simulink model "noisefilterfunction"  (Simulink 7.7)
settings: Solver=ode45  StartTime=0.0  StopTime=1000  RelTol=1e-3
settings Model: Creator=kevin  LastModifiedBy=kevin

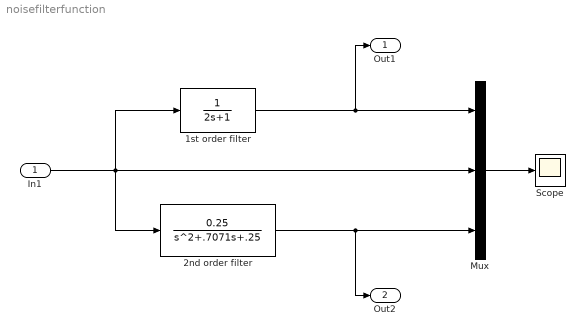
== system noisefilterfunction ==
  In1 : Inport
  1st order filter : TransferFcn  Denominator=[2 1]
  2nd order filter : TransferFcn  Numerator=[0.25]  Denominator=[1 .7071 .25]
  Mux : Mux  Inputs=3
  Scope : Scope
      settings: TimeRange=500  YMin=-4  YMax=4
  Out1 : Outport
  Out2 : Outport  Port=2
  wires:
  2nd order filter/1 -> Mux/3, Out2/1
  1st order filter/1 -> Mux/1, Out1/1
  In1/1 -> Mux/2, 1st order filter/1, 2nd order filter/1
  Mux/1 -> Scope/1
